simulink model "Switch"  (R2016a)
settings: Solver=VariableStepAuto  StartTime=0.0  StopTime=10.0  RelTol=1e-3
settings Model: Creator=hamza  LastModifiedBy=hamza

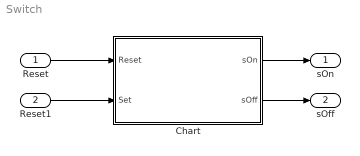
== system Switch ==
  Reset : Inport
  Reset1 : Inport  Port=2
  Chart : Stateflow chart  TreatAsAtomicUnit=on
  sOn : Outport
  sOff : Outport  Port=2
  wires:
  Reset/1 -> Chart/1(Reset)
  Reset1/1 -> Chart/2(Set)
  Chart/1(sOn) -> sOn/1
  Chart/2(sOff) -> sOff/1

== stateflow chart Switch/Chart ==
  state OFF
    entry : sOff = true;
    sOn = false;
  state ON
    entry : sOff = false;
    sOn = true;
  (default) -> OFF
  OFF -> ON : [Set]
  ON -> OFF : [Reset]
  data: Reset input boolean; Set input boolean; sOn output boolean; sOff output boolean
